simulink model "sms_gk_v0"  (R2022b)
settings: Solver=FixedStepAuto  StartTime=0.0  StopTime=10  FixedStep=0.001  RelTol=1e-3
values from neighbouring files (symbols this model uses):
  b = 15    [init.m]
  f = 0.001    [init.m]
  J = 0.0015    [init.m]
  r = 0.75    [init.m]
  rho = 1.2    [init.m]
  s = pi*r^2    (= 1.76714586764)    [init.m]
settings Model: Creator=gkrebs  LastModifiedBy=ZinouAb
settings DebuggingCC: UnconnectedInputMsg=warning  UnconnectedOutputMsg=warning  UnconnectedLineMsg=warning
settings ModelReferenceCC: EnableRefExpFcnMdlSchedulingChecks=on
settings RTWCC: DLArmComputeVersion=19.05

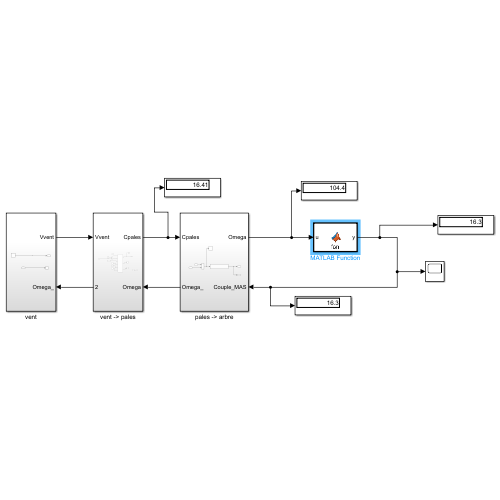
[thumbnail: Simulink's stored preview of the top-level diagram]
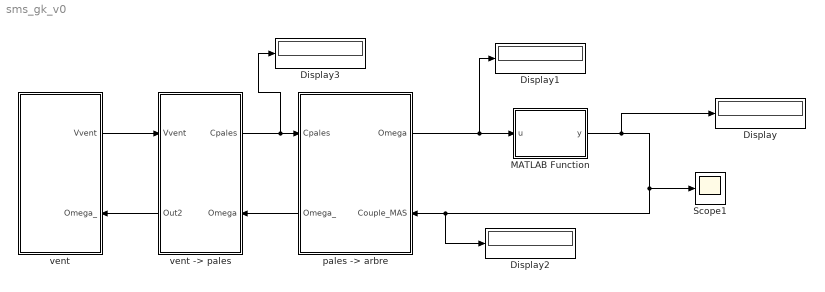
== system sms_gk_v0 ==
  Display{,1..3} (4 alike) : Display
  MATLAB Function : MATLAB Function  TreatAsAtomicUnit=on
  Scope1 : Scope
  "pales -> arbre" : Subsystem
      settings: PortSchema="{\"entries\":[{\"content\":{\"sides\":[{\"content\":{\"connectorIds\":[\"In1\",\"Out2\"]},\"type\":\"ConnectorPlacement.EquallySpacedRectSide\",\"uuid\":\"7b72f56b-829c-42d8-81af-8c3197ae28b8\"},{\"content\":{\"connectorIds\":[\"Out1\",\"In2\"],\"side\":\"RIGHT\"},\"type\":\"ConnectorPlacement.EquallySpacedRectSide\",\"uuid\":\"933a0d6e-d8b0-4587-b5f5-dafea4e8c689\"},{\"content\":{\"connectorIds\":[],\"side\":\"TOP\"},\"type\":\"ConnectorPlacement.EquallySpacedRectSide\",\"uuid\":\"62aafb29-7a9b-464d-894b-b90bef4bbecd\"}]},\"type\":\"ConnectorPlacement.EquallySpacedConnector\",\"uuid\":\"cb6ec811-f3c2-4ea3-9984-69b593c6d991\"}],\"packageUris\":[\"http://schema.mathworks.com/mf0/Connector/R2020b\"],\"version\":\"1.0\"}"
  vent : Subsystem
      settings: PortSchema="{\"entries\":[{\"content\":{\"sides\":[{\"content\":{\"connectorIds\":[]},\"type\":\"ConnectorPlacement.EquallySpacedRectSide\",\"uuid\":\"0e91f94f-7fe4-4cd1-8ec2-e654c3e0b439\"},{\"content\":{\"connectorIds\":[\"Out1\",\"In1\"],\"side\":\"RIGHT\"},\"type\":\"ConnectorPlacement.EquallySpacedRectSide\",\"uuid\":\"94d85fba-6060-45cc-a61d-364af835c548\"},{\"content\":{\"connectorIds\":[],\"side\":\"TOP\"},\"type\":\"ConnectorPlacement.EquallySpacedRectSide\",\"uuid\":\"4fccbcfe-22b7-49b4-8660-9118033fb0d6\"}]},\"type\":\"ConnectorPlacement.EquallySpacedConnector\",\"uuid\":\"5d2980f7-b030-4ec0-b20a-b1940a45daf9\"}],\"packageUris\":[\"http://schema.mathworks.com/mf0/Connector/R2020b\"],\"version\":\"1.0\"}"
  "vent -> pales" : Subsystem
      settings: PortSchema="{\"entries\":[{\"content\":{\"sides\":[{\"content\":{\"connectorIds\":[\"In1\",\"Out2\"]},\"type\":\"ConnectorPlacement.EquallySpacedRectSide\",\"uuid\":\"7b72f56b-829c-42d8-81af-8c3197ae28b8\"},{\"content\":{\"connectorIds\":[\"Out1\",\"In2\"],\"side\":\"RIGHT\"},\"type\":\"ConnectorPlacement.EquallySpacedRectSide\",\"uuid\":\"933a0d6e-d8b0-4587-b5f5-dafea4e8c689\"},{\"content\":{\"connectorIds\":[],\"side\":\"TOP\"},\"type\":\"ConnectorPlacement.EquallySpacedRectSide\",\"uuid\":\"62aafb29-7a9b-464d-894b-b90bef4bbecd\"}]},\"type\":\"ConnectorPlacement.EquallySpacedConnector\",\"uuid\":\"cb6ec811-f3c2-4ea3-9984-69b593c6d991\"}],\"packageUris\":[\"http://schema.mathworks.com/mf0/Connector/R2020b\"],\"version\":\"1.0\"}"
  wires:
  "pales -> arbre"/1(Omega) -> Display1/1, MATLAB Function/1(u)
  "vent -> pales"/1(Cpales) -> Display3/1, "pales -> arbre"/1(Cpales)
  "vent -> pales"/2(Out2) -> vent/1(Omega_)
  "pales -> arbre"/2(Omega_) -> "vent -> pales"/2(Omega)
  MATLAB Function/1(y) -> Display/1, Scope1/1, Display2/1, "pales -> arbre"/2(Couple_MAS)
  vent/1(Vvent) -> "vent -> pales"/1(Vvent)

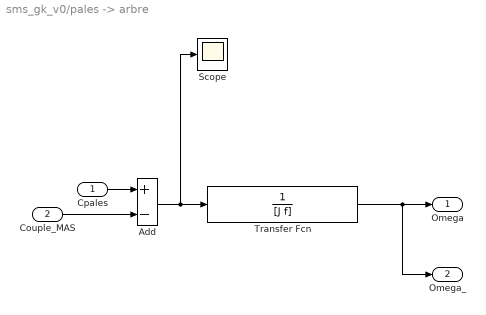
== system sms_gk_v0/pales -> arbre ==
  Cpales : Inport
  Couple_MAS : Inport  Port=2
  Add : Sum  Inputs=+-
  Scope : Scope
  Transfer Fcn : TransferFcn  Denominator=[J f]
  Omega : Outport
  Omega_ : Outport  Port=2
  wires:
  Transfer Fcn/1 -> Omega_/1, Omega/1
  Couple_MAS/1 -> Add/2
  Cpales/1 -> Add/1
  Add/1 -> Scope/1, Transfer Fcn/1

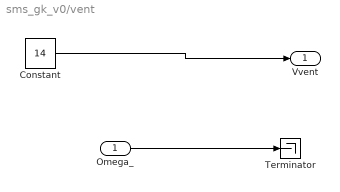
== system sms_gk_v0/vent ==
  Omega_ : Inport
  Constant : Constant  Value=14
  Terminator : Terminator
  Vvent : Outport
  wires:
  Constant/1 -> Vvent/1
  Omega_/1 -> Terminator/1

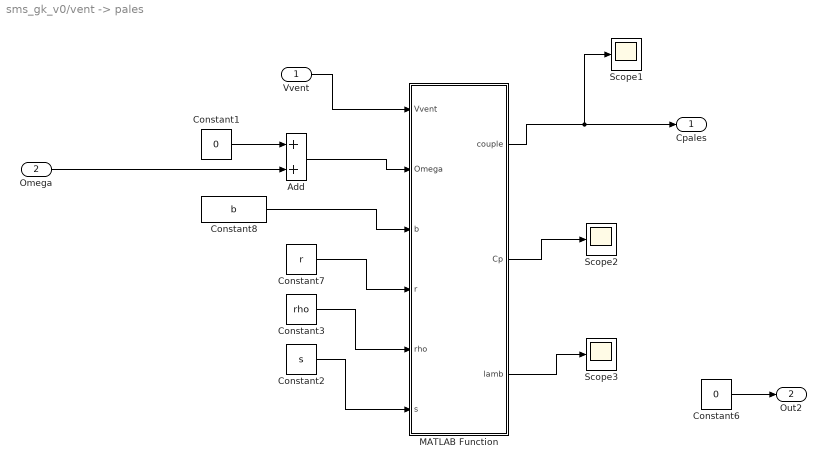
== system sms_gk_v0/vent -> pales ==
  Vvent : Inport
  Omega : Inport  Port=2
  Add : Sum
  Constant1 : Constant  Value=0
  Constant2 : Constant  Value=s
  Constant3 : Constant  Value=rho
  Constant6 : Constant  Value=0
  Constant7 : Constant  Value=r
  Constant8 : Constant  Value=b
  MATLAB Function : MATLAB Function  TreatAsAtomicUnit=on
  Scope1 : Scope
  Scope2 : Scope
  Scope3 : Scope
  Cpales : Outport
  Out2 : Outport  Port=2
  wires:
  Constant6/1 -> Out2/1
  Constant3/1 -> MATLAB Function/5(rho)
  MATLAB Function/1(couple) -> Scope1/1, Cpales/1
  Constant7/1 -> MATLAB Function/4(r)
  Constant8/1 -> MATLAB Function/3(b)
  Vvent/1 -> MATLAB Function/1(Vvent)
  Constant1/1 -> Add/1
  MATLAB Function/2(Cp) -> Scope2/1
  MATLAB Function/3(lamb) -> Scope3/1
  Omega/1 -> Add/2
  Constant2/1 -> MATLAB Function/6(s)
  Add/1 -> MATLAB Function/2(Omega)

== matlab function sms_gk_v0/MATLAB Function ==
  data: u input; y output
function y = fcn(u)

y = 0.0015*u^2-0.00056*u+0.0037;

== matlab function sms_gk_v0/vent -> pales/MATLAB Function ==
  data: Vvent input; couple output; Omega input; b input; r input; rho input; Cp output; lamb output; s input
function [couple,Cp,lamb] = fcn(Vvent,Omega,b,r,rho,s)

    lamb=r*Omega/Vvent;
    if lamb==0    % Pour éviter d'avoir une division par zero par la suite
        lamb=0.001;
    end
        lamb1=1/((1/(lamb+0.089*b))-(0.035/(b^3+1)));
        Cp=0.5*(116/lamb1-0.4*(b-5))*exp(-16.5/lamb1);
        Ct=Cp/lamb;
        couple=0.5*rho*Ct*r*s*Vvent^2;



a=1;
